simulink model "threephase_bucwithmcu_currentcontrol"  (R2021b)
settings: Solver=VariableStepAuto  StartTime=0.0  StopTime=50  RelTol=1e-3
undefined symbols (not defined in the file): Down, Up
libraries: spsDiodeLib x7, spsMeanLib x3, spsVoltageMeasurementLib x2, spsDCMachineLib x1, spsDCVoltageSourceLib x1, spsIGBTLib x1, eePwmGenerator x1, eePowerMeasurement x1, spsSeriesRLCBranchLib x1, spsThreePhaseVIMeasurementLib x1, spsThreePhaseSourceLib x1, spspowerguiLib x1
settings Model: Creator=ASUS  LastModifiedBy=Göktuğ
settings SolverCC: ZeroCrossAlgorithm=Adaptive
settings DebuggingCC: IgnoredZcDiagnostic=none

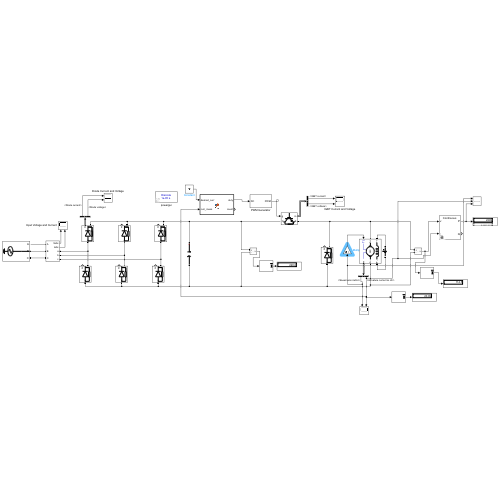
[thumbnail: Simulink's stored preview of the top-level diagram]
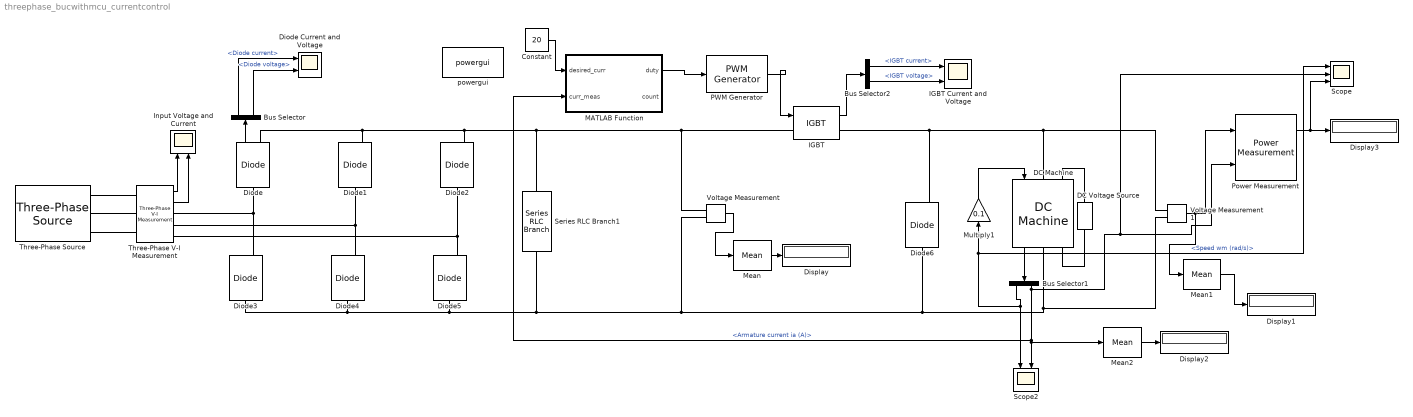
== system threephase_bucwithmcu_currentcontrol ==
  Bus Selector : BusSelector  OutputSignals=Diode current,Diode voltage
  Bus Selector1 : BusSelector  OutputSignals=Speed wm (rad/s),Armature current ia (A)
  Bus Selector2 : BusSelector  OutputSignals=IGBT current,IGBT voltage
  Constant : Constant  Value=20
  DC Machine : spsDCMachineLib/DC Machine  PresetModel=No  MechanicalLoad=Torque TL  FieldType=Wound  ShowDetailedParameters=on  MeasurementBus=off  RLa=[0.8 12.5e-3]  RLf="[ 240  120]"  Laf=1.8  MachineConstant=Torque constant (N.m/A)  Ke=1.8  Kt=1.8  J=1  Bm=0  Tf=0  w0=0  Ifinit=0.62499999938315  TsPowergui=0  TsBlock=-1
  DC Voltage Source : spsDCVoltageSourceLib/DC Voltage Source  Amplitude=150  Measurements=None
  Diode{,1..5} (6 alike) : spsDiodeLib/Diode  Ron=0.001  Lon=0  Vf=0.8  IC=0  UseSnubber=0  Rs=500  Cs=250e-9  Measurements=on
  Diode Current and Voltage : Scope  NumInputPorts=2
  Diode6 : spsDiodeLib/Diode  Ron=0.001  Lon=0  Vf=1.5  IC=0  UseSnubber=0  Rs=500  Cs=250e-9  Measurements=on
  Display{,1..3} (4 alike) : Display
  IGBT : spsIGBTLib/IGBT  Ron=0.001  Lon=0  Vf=1.5  Tf=1e-6  Tt=2e-6  IC=0  Rs=1e5  Cs=inf  Measurements=on
  IGBT Current and Voltage : Scope  NumInputPorts=2
  Input Voltage and Current : Scope  NumInputPorts=2
  MATLAB Function : MATLAB Function  TreatAsAtomicUnit=on
  Mean : spsMeanLib/Mean  Freq=60  Vinit=0  Ts=0
  Mean1 : spsMeanLib/Mean  Freq=60  Vinit=0  Ts=0
  Mean2 : spsMeanLib/Mean  Freq=60  Vinit=0  Ts=0
  Multiply1 : Gain  Gain=0.1
  PWM Generator : eePwmGenerator/PWM Generator  CarrCount=Up-Down  Tper=5e-5  Tdelay=0  Ts=0
  Power Measurement : eePowerMeasurement/Power Measurement  LabelModeActiveChoice=Continuous  F=60  K=[0 1 2 3]  Ts=0
      settings: SourceProductBaseCode=PS
  Scope : Scope  NumInputPorts=3
  Scope2 : Scope  NumInputPorts=2
  Series RLC Branch1 : spsSeriesRLCBranchLib/Series RLC Branch  LConnTagsString=__new0  RConnTagsString=__new0  BranchType=C  Resistance=0.000002  Inductance=1e-3  SetiL0=off  InitialCurrent=0  Capacitance=470e-6  Setx0=off  InitialVoltage=0  Measurements=None
  Three-Phase V-I Measurement : spsThreePhaseVIMeasurementLib/Three-Phase V-I Measurement  VoltageMeasurement=phase-to-ground  SetLabelV=off  LabelV=Vabc  Vpu=off  VpuLL=off  CurrentMeasurement=yes  SetLabelI=off  LabelI=Iabc  Ipu=off  Pbase=100e6  Vbase=500e3  OutputType=Complex  PhasorSimulation=off  PSBequivalent=0
  Three-Phase Source : spsThreePhaseSourceLib/Three-Phase Source  InternalConnection=Yg  VoltagePhases=off  Voltage=170  PhaseAngle=0  Voltage_phases=[25e3 25e3 25e3]/sqrt(3)  PhaseAngles_phases=[0 -120 +120]  Frequency=50  NonIdealSource=off  SpecifyImpedance=off  Resistance=0.8929  Inductance=16.58e-3  ShortCircuitLevel=100e6  BaseVoltage=25e3  XRratio=7  BusType=swing  Pref=10e3  Qref=0  Prefabc=[10e3, 10e3, 10e3]  Qrefabc=[0, 0, 0]  Qmin=-inf  Qmax=inf
  Voltage Measurement : spsVoltageMeasurementLib/Voltage Measurement  PhasorSimulation=off  OutputType=Complex  PSBequivalent=0
  Voltage Measurement1 : spsVoltageMeasurementLib/Voltage Measurement  PhasorSimulation=off  OutputType=Complex  PSBequivalent=0
  powergui : spspowerguiLib/powergui  Priority=1  SimulationMode=Discrete  SampleTime=10e-6  frequency=60  Iterations=50  frequencyindice=50  Pbase=100e6  ErrMax=1e-4  UnitsV=kV  UnitsW=MW  buscounter=0  FunctionMessages=off  echomessages=off  EnableUseOfTLC=off  CurrentSourceSwitches=off  DisableSnubberDevices=off  DisableRonSwitches=off  DisableVfSwitches=off  DisplayEquations=off  AutomaticDiscreteSolvers=off  SolverType=Tustin/Backward Euler (TBE)  Interpol=off  ExternalGateDelay=off  methode=off  Ts=100  x0status=blocks  SPID=on  SwTol=0  HookPort=off  NonlinearTolerance=1e-4  nMaxIteration=100  ContinueOnMaxIteration=off  RestoreLinks=warning  ResistiveCurrentMeasurement=off  Frange=[0:2:500]  Ylog=off  Xlog=on  ShowGrid=off  save=off  variable=ZData  structure=0  ZoomFFT=off  StartTime=0.0  cycles=1  DisplayStyle=1  fundamental=60  FreqAxis=off  MaxFrequency=1000  frequencyindicesteady=1  RmsSteady=1  display=off
  wires:
  Voltage Measurement/1 -> Mean/1
  Mean/1 -> Display/1
  Diode/1 -> Bus Selector/1
  Bus Selector/1 -> Diode Current and Voltage/1  "<Diode current>"
  Bus Selector/2 -> Diode Current and Voltage/2  "<Diode voltage>"
  PWM Generator/1 -> IGBT/1
  DC Machine/1 -> Bus Selector1/1
  Bus Selector1/2 -> Scope/2, Power Measurement/2, Scope2/2, Mean2/1, MATLAB Function/2(curr_meas)  "<Armature current ia (A)>"
  Voltage Measurement1/1 -> Power Measurement/1, Mean1/1
  Mean1/1 -> Display1/1
  Three-Phase V-I Measurement/1 -> Input Voltage and Current/1
  Three-Phase V-I Measurement/2 -> Input Voltage and Current/2
  IGBT/1 -> Bus Selector2/1
  Bus Selector2/1 -> IGBT Current and Voltage/1  "<IGBT current>"
  Bus Selector2/2 -> IGBT Current and Voltage/2  "<IGBT voltage>"
  Mean2/1 -> Display2/1
  Multiply1/1 -> DC Machine/1
  Bus Selector1/1 -> Scope/1, Multiply1/1, Scope2/1  "<Speed wm (rad/s)>"
  MATLAB Function/1(duty) -> PWM Generator/1
  Constant/1 -> MATLAB Function/1(desired_curr)
  Power Measurement/1 -> Scope/3, Display3/1
  connections:
  Diode5/RConn1 -- Three-Phase V-I Measurement/RConn3 -- Diode2/LConn1
  Diode4/RConn1 -- Three-Phase V-I Measurement/RConn2 -- Diode1/LConn1
  Diode3/RConn1 -- Three-Phase V-I Measurement/RConn1 -- Diode/LConn1
  Three-Phase V-I Measurement/LConn1 -- Three-Phase Source/RConn1
  Three-Phase Source/RConn2 -- Three-Phase V-I Measurement/LConn2
  Three-Phase Source/RConn3 -- Three-Phase V-I Measurement/LConn3
  Diode3/LConn1 -- Series RLC Branch1/RConn1 -- Diode6/LConn1 -- DC Machine/RConn1 -- Voltage Measurement1/LConn2 -- Voltage Measurement/LConn2 -- Diode5/LConn1 -- Diode4/LConn1
  Diode1/RConn1 -- Voltage Measurement/LConn1 -- IGBT/LConn1 -- Series RLC Branch1/LConn1 -- Diode2/RConn1 -- Diode/RConn1
  IGBT/RConn1 -- DC Machine/LConn1 -- Voltage Measurement1/LConn1 -- Diode6/RConn1
  DC Machine/LConn2 -- DC Voltage Source/RConn1
  DC Machine/RConn2 -- DC Voltage Source/LConn1

== matlab function threephase_bucwithmcu_currentcontrol/MATLAB Function ==
  settings: updateMethod=DISCRETE  sampleTime=10e-6
  data: desired_curr input; duty output; curr_meas input; count output
function [duty, count]= fcn(desired_curr, curr_meas)
persistent tick
persistent calcduty
persistent integral
if(isempty(tick))
    tick=0;
end
if(isempty(calcduty))
    calcduty=0;
end
if(isempty(integral))
    integral=-0.5;
end

if(tick == 0)
    integral = integral + (desired_curr-curr_meas)/10;
    if(integral<-0.6)
        integral = -0.6;
    elseif(integral>0.6)
        integral = 0.6;
    end
    calcduty = (desired_curr-curr_meas)*0.5+integral;
    if(desired_curr>curr_meas)
        calcduty = calcduty+0.0001;
    elseif(desired_curr<curr_meas)
        calcduty = calcduty-0.0001;
    end
end
tick = tick + 1;

if(tick==10) 
    tick = 0;
end

if(calcduty>1)
    calcduty = 1;
elseif(calcduty<0)
    calcduty=0;
end
count = tick;
duty = calcduty;
end
